simulink model "TestLogOptoforce"  (R2017b)
settings: Solver=FixedStepDiscrete  StartTime=0.0  StopTime=inf  FixedStep=0.02  RelTol=1e-3  EnableMultiTasking=on
undefined symbols (not defined in the file or in its folder): serial
libraries: etargetslib x2, instrumentlib x2
settings Model: Creator=mine  LastModifiedBy=BCI-USER
settings DataIOCC: LimitDataPoints=on  SaveFormat=Array
settings OptimizationCC: LifeSpan=inf
settings DebuggingCC: UnderspecifiedInitializationDetection=Classic  MergeDetectMultiDrivingBlocksExec=none  SolverPrmCheckMsg=warning  StateNameClashWarn=warning  SFUnexpectedBacktrackingDiag=warning  SFNoUnconditionalDefaultTransitionDiag=warning  SFExecutionAtInitializationDiag=none
settings HardwareCC: ProdBitPerPointer=32  ProdBitPerSizeT=32  ProdBitPerPtrDiffT=32  ProdLargestAtomicFloat=None  ProdIntDivRoundTo=Undefined  ProdEndianess=Unspecified  ProdWordSize=32  ProdHWDeviceType=32-bit Generic
settings ModelReferenceCC: PropagateSignalLabelsOutOfModel=off
settings CodeAppCC: StateflowObjectComments=on
settings GRTTargetCC: TargetLangStandard=C89/C90 (ANSI)  GeneratePreprocessorConditionals=Disable all
settings ConfigComp: CovMetricSettings=dw  CovHtmlReporting=on  CovSaveCumulativeToWorkspaceVar=on  CovSaveSingleToWorkspaceVar=on  CovExternalEMLEnable=off

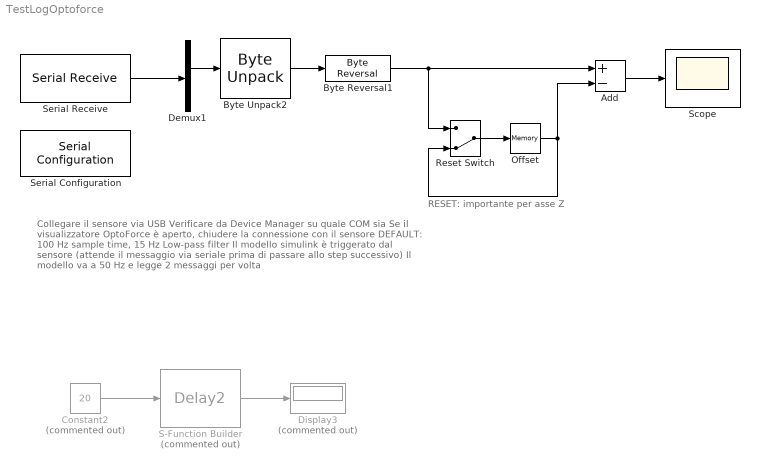
== system TestLogOptoforce ==
  note: RESET: importante per asse Z
  note: Collegare il sensore via USB
      | Verificare da Device Manager su quale COM sia
      | Se il visualizzatore OptoForce è aperto, chiudere la connessione con il sensore
      |
      | DEFAULT: 100 Hz sample time, 15 Hz Low-pass filter
      |
      | Il modello simulink è triggerato dal sensore
      | (attende il messaggio via seriale prima di passare allo step successivo)
      | Il modello va a 50 Hz e legge 2 messaggi per volta
  Add : Sum  Inputs=+-
  Byte Reversal1 : etargetslib/Byte Reversal  numInp=1
  Byte Unpack2 : etargetslib/Byte Unpack  dimensions={3}  datatypes={'int16'}  byteAlign=1
  Constant2 : Constant  Commented=on  Value=20  OutDataTypeStr=uint32  SampleTime=-1
  Demux1 : Demux  Outputs="[3 6 20  29]"
  Display3 : Display  Commented=on
  Offset : Memory  InitialCondition=[0 0 0]
  Reset Switch : ManualSwitch  CurrentSetting=0
  S-Function Builder : S-Function  Commented=on  InitFcn=try, set_param(gcb,'FunctionName','Delay2'), end  FunctionName=Delay2  SFunctionModules=Delay2_wrapper  SFunctionDeploymentMode=off  EnableBusSupport=off  mask(S-Function Builder){}
      mask help: Simulink:masks:SFunctionBuilder_MD
      mask init:
      | val = [[.9  0.75 0.75 1 1 .9 .9 1]',[1 1 0.75 0.75 .9 .9 1 .9]'];try , sys = get_param(gcb,'SfunBuilderFcnName');if isempty(sys), sys = get_param(gcb,'FunctionName'); end,catch, sys = get_param(gcb,'FunctionName'); end
      settings: CopyFcn=set_param(gcbh,'LinkStatus','none')  PreSaveFcn=try, set_param(gcb,'FunctionName','Delay2'), end  OpenFcn=sfunctionwizard(gcbh)
      mask Display: plot(val(:,1),val(:,2)),disp(sys), port_label('input',1,'u0'), port_label('output',1,'y0')
  Scope : Scope
  Serial Configuration : instrumentlib/Serial Configuration  Priority=-200000  ComPortMenu=<Please select a port...>  ComPort=COM2  ObjConstructor=serial('COM2');  BaudRate=115200  DataBits=8  Parity=none  StopBits=1  FlowControl=none  Timeout=5  ByteOrder=LittleEndian
  Serial Receive : instrumentlib/Serial Receive  ComPortMenu=<Please select a port...>  ComPort=COM2  ObjConstructor=serial('COM2');  Terminator=<none>  DataSize="[58   1]"  DataType=uint8  EnableBlockingMode=on  ActionDataUnavailable=Output last received value  CustomValue=0  SampleTime=-1
  wires:
  Constant2/1 -> S-Function Builder/1
  S-Function Builder/1 -> Display3/1
  Serial Receive/1 -> Demux1/1
  Byte Unpack2/1 -> Byte Reversal1/1
  Demux1/2 -> Byte Unpack2/1
  Byte Reversal1/1 -> Reset Switch/1, Add/1
  Add/1 -> Scope/1
  Reset Switch/1 -> Offset/1
  Offset/1 -> Reset Switch/2, Add/2
